simulink model "baohanfenglunzhikuai"  (Simulink 7.4)
settings: Solver=ode45  StartTime=0.0  StopTime=0.1  RelTol=1e-6  AbsTol=1e-6
libraries: powerlib x3
settings Model: Creator=Administrator  LastModifiedBy=Administrator

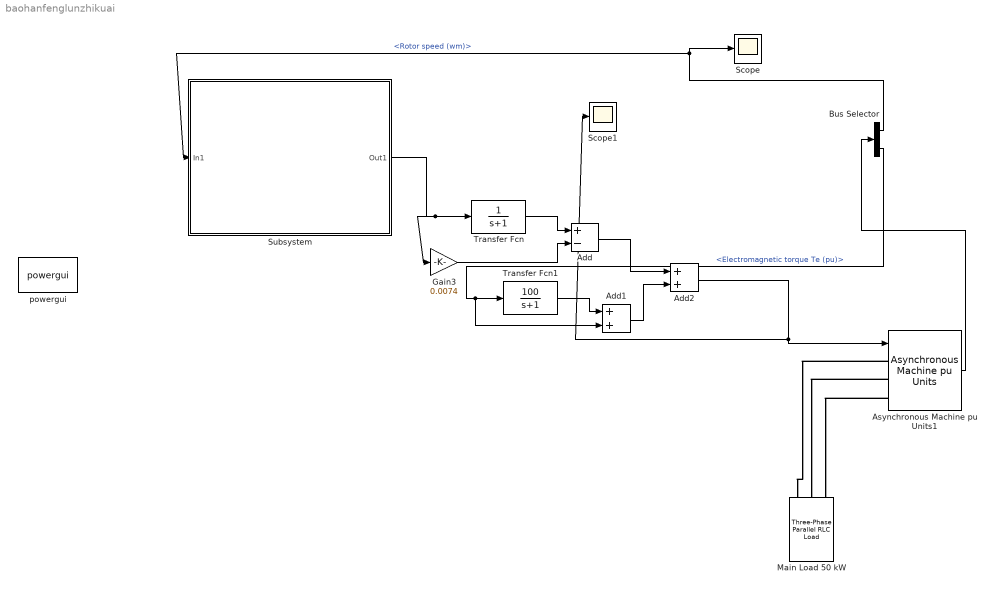
== system baohanfenglunzhikuai ==
  Add : Sum  Inputs=+-  OutDataType=fixdt(1, 16)  OutScaling=2^-10
  Add1 : Sum  OutDataType=fixdt(1, 16)  OutScaling=2^-10
  Add2 : Sum  OutDataType=fixdt(1, 16)  OutScaling=2^-10
  Asynchronous Machine pu Units1 : powerlib/Machines/Asynchronous Machine pu Units  DialogController=POWERSYS.PowerSysDialog  SystemSampleTime=-1  PresetModel=No  MechanicalLoad=Torque Tm  ShowDetailedParameters=on  RotorType=Squirrel-cage  ReferenceFrame=Rotor  NominalParameters=[3730 460 50]  Stator=[0.01965 0.0397]  Rotor=[0.01909 0.0397]  Lm=1.354  Mechanical=[0.09526 0.05479 2]  PolePairs=2  InitialConditions="[ 1,0   0,0,0   0,0,0 ]"  Units=pu  LoadFlowParameters=0  SimulateSaturation=off  Saturation="[0.212,0.4201,0.8125,1.0979,1.4799,2.2457,3.2586,4.5763,6.4763 ;   0.5,0.7,0.9,1,1.1,1.2 ,1.3,1.4,1.5]"  TsPowergui=0  TsBlock=-1  IterativeModel=Forward Euler
  Bus Selector : BusSelector  OutputSignals=Mechanical.Rotor speed (wm),Mechanical.Electromagnetic torque Te (pu)
  Gain3 : Gain  Gain=0.0074  ParameterDataType=fixdt(1, 16)  ParameterScaling=2^0  OutDataType=fixdt(1, 16)  OutScaling=2^0
  Main Load 50 kW : powerlib/Elements/Three-Phase Parallel RLC Load  DialogController=POWERSYS.PowerSysDialog  PhysicalDomain=powersysdomain  SubClassName=unknown  LeftPortType=p1  RightPortType=p1  LConnTagsString=A|B|C  Configuration=Y (grounded)  NominalVoltage=460  NominalFrequency=50  ActivePower=50e3  InductivePower=0  CapacitivePower=0  Measurements=None
  Scope : Scope
      settings: TimeRange=1  YMin=-1  YMax=1
  Scope1 : Scope
      settings: TimeRange=10  YMin=-4.5e+066  YMax=0
  Subsystem : Subsystem
  Transfer Fcn : TransferFcn  Denominator=[1 1]  AbsoluteTolerance=0.001
  Transfer Fcn1 : TransferFcn  Numerator=[100]  Denominator=[1 1]
  powergui : powerlib/powergui  Priority=1  SystemSampleTime=-1  SimulationMode=Discrete  SampleTime=1e-6  frequency=60  SPID=off  DisableSnubberDevices=off  DisableRonSwitches=off  DisableVfSwitches=off  SwTol=0  Interpol=off  frequencyindice=50  echomessages=off  HookPort=off  DisplayEquations=off  FunctionMessages=off  EnableUseOfTLC=off  x0status=blocks  RestoreLinks=warning  Frange=[0:2:500]  Ylog=off  Xlog=on  ShowGrid=off  save=off  variable=ZData  ZoomFFT=on  StartTime=0.0  cycles=1  DisplayStyle=1  fundamental=60  FreqAxis=off  MaxFrequency=1000  frequencyindicesteady=1  RmsSteady=1  display=off  Ts=0  methode=off
  wires:
  Asynchronous Machine pu Units1/1 -> Bus Selector/1
  Bus Selector/1 -> Scope/1, Subsystem/1(In1)  "<Rotor speed (wm)>"
  Transfer Fcn/1 -> Add/1
  Subsystem/1(Out1) -> Transfer Fcn/1, Gain3/1
  Transfer Fcn1/1 -> Add1/1
  Add/1 -> Add2/1
  Add1/1 -> Add2/2
  Bus Selector/2 -> Transfer Fcn1/1, Add1/2  "<Electromagnetic torque Te (pu)>"
  Add2/1 -> Asynchronous Machine pu Units1/1, Scope1/1
  Gain3/1 -> Add/2
  connections:
  Asynchronous Machine pu Units1/LConn1 -- Main Load 50 kW/LConn1
  Asynchronous Machine pu Units1/LConn2 -- Main Load 50 kW/LConn2
  Asynchronous Machine pu Units1/LConn3 -- Main Load 50 kW/LConn3

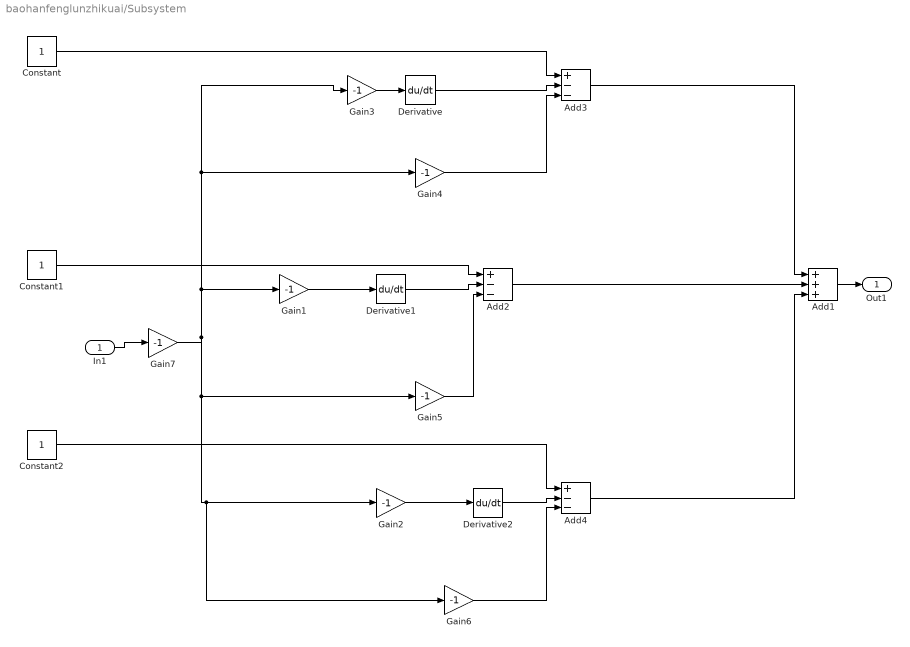
== system baohanfenglunzhikuai/Subsystem ==
  In1 : Inport  OutDataType=fixdt(1, 16)  OutScaling=2^0
  Add1 : Sum  Inputs=+++  OutDataType=fixdt(1, 16)  OutScaling=2^-10
  Add2 : Sum  Inputs=+--  OutDataType=fixdt(1, 16)  OutScaling=2^-10
  Add3 : Sum  Inputs=+--  OutDataType=fixdt(1, 16)  OutScaling=2^-10
  Add4 : Sum  Inputs=+--  OutDataType=fixdt(1, 16)  OutScaling=2^-10
  Constant : Constant  OutDataType=fixdt(1, 16)  OutScaling=2^0
  Constant1 : Constant  OutDataType=fixdt(1, 16)  OutScaling=2^0
  Constant2 : Constant  OutDataType=fixdt(1, 16)  OutScaling=2^0
  Derivative : Derivative
  Derivative1 : Derivative
  Derivative2 : Derivative
  Gain{1..7} (7 alike) : Gain  Gain=-1  ParameterDataType=fixdt(1, 16)  ParameterScaling=2^0  OutDataType=fixdt(1, 16)  OutScaling=2^0
  Out1 : Outport
  wires:
  Add3/1 -> Add1/1
  Add4/1 -> Add1/3
  Gain3/1 -> Derivative/1
  Derivative/1 -> Add3/2
  Gain1/1 -> Derivative1/1
  Derivative1/1 -> Add2/2
  Gain2/1 -> Derivative2/1
  Derivative2/1 -> Add4/2
  Add2/1 -> Add1/2
  Gain4/1 -> Add3/3
  Gain5/1 -> Add2/3
  Gain6/1 -> Add4/3
  Constant/1 -> Add3/1
  Constant1/1 -> Add2/1
  Constant2/1 -> Add4/1
  Add1/1 -> Out1/1
  Gain7/1 -> Gain1/1, Gain3/1, Gain4/1, Gain5/1, Gain2/1, Gain6/1
  In1/1 -> Gain7/1
